simulink model "shoot4"  (R2017b)
settings: Solver=VariableStepAuto  StartTime=0.0  StopTime=10.0  RelTol=1e-3
settings Model: Creator=ghleila  LastModifiedBy=ghleila

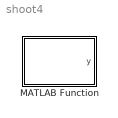
== system shoot4 ==
  MATLAB Function : MATLAB Function  TreatAsAtomicUnit=on

== matlab function shoot4/MATLAB Function ==
  data: y output
function y = fcn

global u

u=u+2;
y = u;
